simulink model "Test_du_despoire_Gcm"  (R2024a)
settings: Solver=FixedStepAuto  StartTime=0.0  StopTime=10.0  RelTol=1e-3
settings Model: Creator=levm1106  LastModifiedBy=levm1106

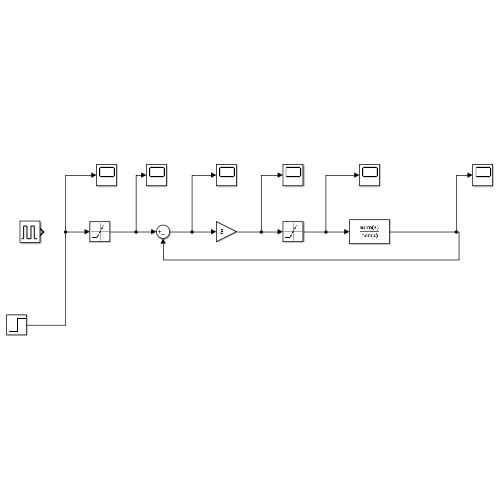
[thumbnail: Simulink's stored preview of the top-level diagram]
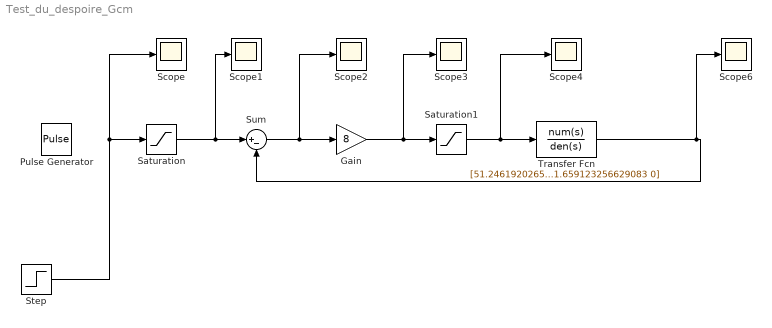
== system Test_du_despoire_Gcm ==
  Gain : Gain  Gain=8
  Pulse Generator : DiscretePulseGenerator  PulseType=Time based  Amplitude=pi/6  Period=5  PulseWidth=5
  Saturation : Saturate  UpperLimit=0.9974  LowerLimit=-0.9974
  Saturation1 : Saturate  UpperLimit=10  LowerLimit=-10
  Scope{,1..4,6} (6 alike) : Scope
  Step : Step  Time=0  Before=pi/6  After=pi/6  SampleTime=0.01
  Sum : Sum  Inputs=|+-
  Transfer Fcn : TransferFcn  Numerator=[51.246192026592354]  Denominator=[1 31.659123256629083 0]
  wires:
  Saturation/1 -> Scope1/1, Sum/1
  Sum/1 -> Scope2/1, Gain/1
  Gain/1 -> Scope3/1, Saturation1/1
  Saturation1/1 -> Scope4/1, Transfer Fcn/1
  Transfer Fcn/1 -> Scope6/1, Sum/2
  Step/1 -> Scope/1, Saturation/1
